simulink model "EKF_Sim_FAEKF"  (R2018a)
settings: Solver=ode4  StartTime=time_start  StopTime=time_end  FixedStep=time_step  MaxStep=0.1  RelTol=1e-6  AbsTol=1e-6
values from neighbouring files (symbols this model uses):
  FUZZY_props =     [FAEKF_FuzzyProps.mat]    (also in FFNAV_FAEKF_RunSim.m = FFNAV_FAEKF_FuzzyInitialize(MSFplot_flag))
  GPS_r_STD = 10*GPS_r_STD    [FFNAV_FAEKF_RunSim.m]
  GPS_v_STD = 10*GPS_v_STD    [FFNAV_FAEKF_RunSim.m]
  N_window = 30    [FFNAV_FAEKF_RunSim.m]
  Q0 = 10*Q0    [FFNAV_FAEKF_RunSim.m]
  Q_adapt = Q0    [FFNAV_FAEKF_FuzzyAdapt.m]    (also in FFNAV_FAEKF_RunSim.m = 0)
  R0 = R0    [FFNAV_FAEKF_RunSim.m]
  R_adapt = R0*beta^(-2*(k))    [FFNAV_FAEKF_FuzzyAdapt.m]    (also in FFNAV_FAEKF_RunSim.m = 0)
  time_step = 1    [FFNAV_FAEKF_RunSim.m]
undefined symbols (not defined in the file or in its folder): COE_chaser, COE_target, Constants, mu, n, PropOptions_chaser, PropOptions_target, theta0_target
libraries: dspindex x9, dspstat3 x7, dspmtrx3 x1
(part 1 of 2)
settings Model: Creator=corytfraser  LastModifiedBy=Cory
settings SolverCC: AutoScaleAbsTol=off
settings DataIOCC: LimitDataPoints=on  SaveFormat=Array  SignalLoggingSaveFormat=ModelDataLogs
settings OptimizationCC: BlockReduction=off  BooleanDataType=off  ExpressionDepthLimit=2147483647  LifeSpan=inf
settings DebuggingCC: SaveWithParameterizedLinksMsg=none  UnderspecifiedInitializationDetection=Classic  MergeDetectMultiDrivingBlocksExec=none  MultiTaskDSMMsg=warning  MultiTaskCondExecSysMsg=none  FcnCallInpInsideContextMsg=warning  AllowSymbolicDim=off  StateNameClashWarn=warning  SFUnexpectedBacktrackingDiag=warning  SFNoUnconditionalDefaultTransitionDiag=warning  SFExecutionAtInitializationDiag=none
settings HardwareCC: ProdBitPerPointer=32  ProdBitPerSizeT=32  ProdBitPerPtrDiffT=32  ProdLargestAtomicFloat=None  ProdIntDivRoundTo=Undefined  ProdEndianess=Unspecified  ProdWordSize=32  ProdHWDeviceType=32-bit Generic  TargetUnknown=on
settings ModelReferenceCC: PropagateSignalLabelsOutOfModel=off
settings CodeAppCC: StateflowObjectComments=on
settings GRTTargetCC: TargetLangStandard=C89/C90 (ANSI)  GeneratePreprocessorConditionals=Disable all
settings ConfigComp: CovMetricSettings=dw  CovHtmlReporting=on  CovSaveCumulativeToWorkspaceVar=on  CovSaveSingleToWorkspaceVar=on  CovExternalEMLEnable=off  CovSFcnEnable=off

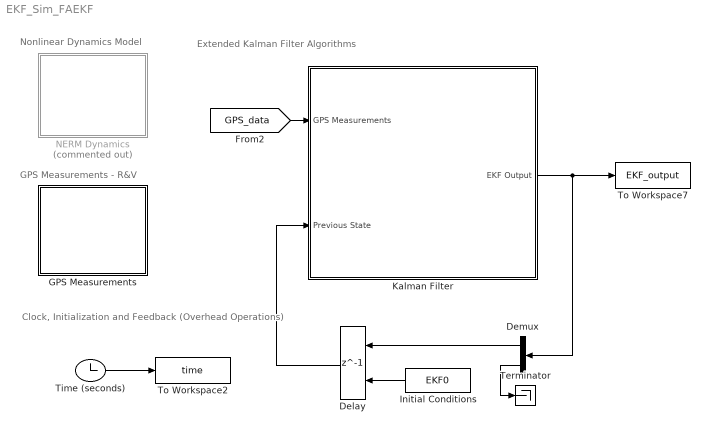
== system EKF_Sim_FAEKF ==
  note: Clock, Initialization and Feedback
      |         (Overhead Operations)
  note: Extended Kalman Filter
      |          Algorithms
  note: GPS Measurements - R&V
  note: Nonlinear Dynamics Model
  Delay : Delay  DelayLength=1  InitialConditionSource=Input port  InitialCondition=0  SampleTime=time_step
      settings: InputPortMap=u0,p4
  Demux : Demux  Outputs=[117 -1]
  "GPS Measurements " : Subsystem
      mask Display: image('C:\Users\Cory\OneDrive\FFNAV Project\MATLAB Code\NERM EKF Simulation\Masks\GPS Image.jpg');
  Initial Conditions : FromWorkspace  VariableName=EKF0  SampleTime=time_step
  Kalman Filter : Subsystem  Variant=on
  NERM Dynamics : Subsystem  Commented=on
      mask Display: image('C:\Users\Cory\OneDrive\FFNAV Project\MATLAB Code\NERM EKF Simulation\Masks\Proba-3.jpg');
  Terminator : Terminator
  Time (seconds) : Clock
      settings: Decimation=1000
  To Workspace2 : ToWorkspace  VariableName=time  SampleTime=-1
  To Workspace7 : ToWorkspace  VariableName=EKF_output  SampleTime=-1
  wires:
  Time (seconds)/1 -> To Workspace2/1
  Kalman Filter/1(EKF Output) -> Demux/1, To Workspace7/1
  Initial Conditions/1 -> Delay/2
  Delay/1 -> Kalman Filter/2(Previous State)
  [GPS_data] -> Kalman Filter/1(GPS Measurements)
  Demux/2 -> Terminator/1
  Demux/1 -> Delay/1

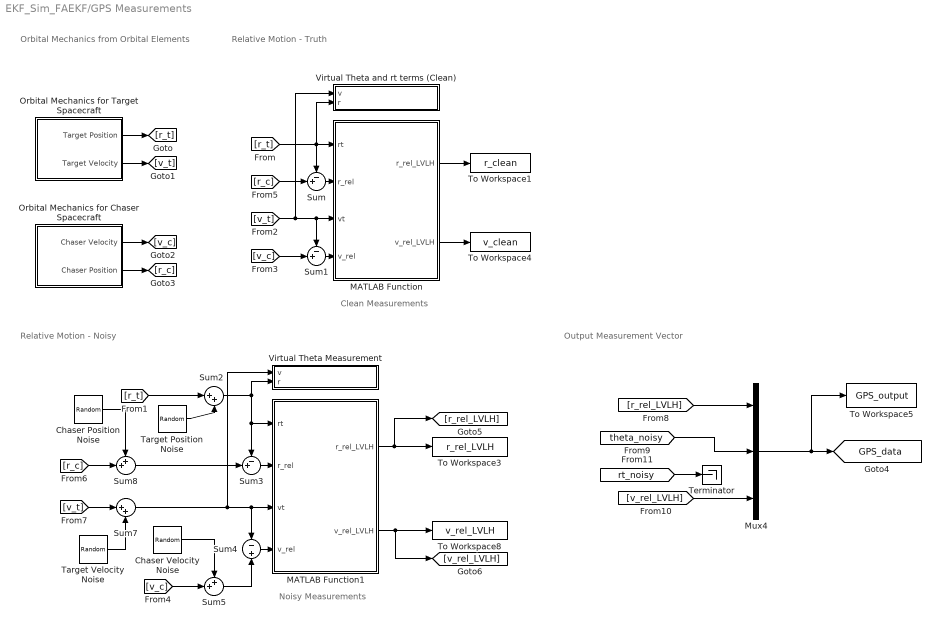
== system EKF_Sim_FAEKF/GPS Measurements  ==
  note: Output Measurement Vector
  note: Relative Motion - Noisy
  note: Relative Motion - Truth
  note: Orbital Mechanics
      | from Orbital Elements
  note: Noisy Measurements
  note: Clean Measurements
  Chaser Position Noise : RandomNumber  Variance=GPS_r_STD^2  Seed=1222  SampleTime=time_step
  Chaser Velocity Noise : RandomNumber  Variance=GPS_v_STD^2  Seed=99999999  SampleTime=time_step
  MATLAB Function : MATLAB Function  TreatAsAtomicUnit=on
  MATLAB Function1 : MATLAB Function  TreatAsAtomicUnit=on
  Mux4 : Mux  Inputs=3
  Orbital Mechanics for Target Spacecraft : Subsystem
  Orbital Mechanics for Chaser Spacecraft : Subsystem
  Sum : Sum  Inputs=-+|
  Sum1 : Sum  Inputs=-+|
  Sum2 : Sum  Inputs=|++
  Sum3 : Sum  Inputs=-+|
  Sum4 : Sum  Inputs=-|+
  Sum5 : Sum  Inputs=++|
  Sum7 : Sum  Inputs=|++
  Sum8 : Sum  Inputs=++|
  Target Position Noise : RandomNumber  Variance=GPS_r_STD^2  Seed=999  SampleTime=time_step
  Target Velocity Noise : RandomNumber  Variance=GPS_v_STD^2  Seed=2000  SampleTime=time_step
  Terminator : Terminator
  To Workspace1 : ToWorkspace  VariableName=r_clean  SampleTime=-1
  To Workspace3 : ToWorkspace  VariableName=r_rel_LVLH  SampleTime=-1
  To Workspace4 : ToWorkspace  VariableName=v_clean  SampleTime=-1
  To Workspace5 : ToWorkspace  VariableName=GPS_output  SampleTime=-1
  To Workspace8 : ToWorkspace  VariableName=v_rel_LVLH  SampleTime=-1
  Virtual Theta Measurement : Subsystem
  Virtual Theta and rt terms (Clean) : Subsystem
  tag scope: GPS_data=global
  wires:
  Orbital Mechanics for Target Spacecraft/1(Target Position) -> [r_t]
  Sum/1 -> MATLAB Function/2(r_rel)
  Sum1/1 -> MATLAB Function/4(v_rel)
  MATLAB Function/2(v_rel_LVLH) -> To Workspace4/1
  MATLAB Function/1(r_rel_LVLH) -> To Workspace1/1
  Mux4/1 -> To Workspace5/1, [GPS_data]
  MATLAB Function1/2(v_rel_LVLH) -> [v_rel_LVLH], To Workspace8/1
  MATLAB Function1/1(r_rel_LVLH) -> [r_rel_LVLH], To Workspace3/1
  Sum7/1 -> Virtual Theta Measurement/1(v), MATLAB Function1/3(vt), Sum4/1
  Sum3/1 -> MATLAB Function1/2(r_rel)
  Sum4/1 -> MATLAB Function1/4(v_rel)
  Sum5/1 -> Sum4/2
  Sum8/1 -> Sum3/2
  [r_t] -> Virtual Theta and rt terms (Clean)/2(r), Sum/1, MATLAB Function/1(rt)
  [v_t] -> Sum1/1, MATLAB Function/3(vt), Virtual Theta and rt terms (Clean)/1(v)
  [v_c] -> Sum1/2
  Orbital Mechanics for Chaser Spacecraft/1(Chaser Velocity) -> [v_c]
  [r_c] -> Sum/2
  Orbital Mechanics for Chaser Spacecraft/2(Chaser Position) -> [r_c]
  Orbital Mechanics for Target Spacecraft/2(Target Velocity) -> [v_t]
  [r_t] -> Sum2/1
  [r_c] -> Sum8/2
  [v_t] -> Sum7/1
  [v_c] -> Sum5/2
  Sum2/1 -> MATLAB Function1/1(rt), Sum3/1, Virtual Theta Measurement/2(r)
  Chaser Position Noise/1 -> Sum8/1
  Target Position Noise/1 -> Sum2/2
  Target Velocity Noise/1 -> Sum7/2
  Chaser Velocity Noise/1 -> Sum5/1
  [r_rel_LVLH] -> Mux4/1
  [v_rel_LVLH] -> Mux4/3
  [theta_noisy] -> Mux4/2
  [rt_noisy] -> Terminator/1

== system EKF_Sim_FAEKF/Kalman Filter ==
  GPS Measurements : Inport
  Previous State : Inport  Port=2
  EKF : Subsystem  VariantControl=EKF_flag == 0
  FAEKF : Subsystem  VariantControl=EKF_flag == 2
  MLE-EKF : Subsystem  VariantControl=EKF_flag == 1
  EKF Output : Outport

== system EKF_Sim_FAEKF/NERM Dynamics ==
  Demux : Demux  Outputs=[10 -1]
  Demux1 : Demux  Outputs=10
  Initial Conditions : FromWorkspace  VariableName=EKF0  SampleTime=time_step
  Mux : Mux  Inputs=10
  NERM Propagation : Subsystem
  Terminator1 : Terminator
  To Workspace6 : ToWorkspace  VariableName=NERM_output  SampleTime=-1
  wires:
  Demux1/9 -> NERM Propagation/9(theta_dot0)
  Demux1/6 -> NERM Propagation/6(x_dot0_chaser)
  Demux1/4 -> NERM Propagation/4(theta0_target)
  Demux1/3 -> NERM Propagation/3(z0_chaser)
  Initial Conditions/1 -> Demux/1
  Demux1/7 -> NERM Propagation/7(y_dot0_chaser)
  Demux1/2 -> NERM Propagation/2(y0_chaser)
  Demux1/1 -> NERM Propagation/1(x0_chaser)
  NERM Propagation/1(x) -> Mux/1
  NERM Propagation/2(y) -> Mux/2
  NERM Propagation/3(z) -> Mux/3
  Demux/1 -> Demux1/1  "Initial  State Vector"
  NERM Propagation/7(y_dot) -> Mux/7
  NERM Propagation/4(theta_target) -> Mux/4
  NERM Propagation/9(theta_dot_target) -> Mux/9
  NERM Propagation/10(rt_dot) -> Mux/10
  NERM Propagation/6(x_dot) -> Mux/6
  NERM Propagation/8(z_dot) -> Mux/8
  NERM Propagation/5(rt) -> Mux/5
  Demux1/8 -> NERM Propagation/8(z_dot0_chaser)
  Mux/1 -> To Workspace6/1
  Demux/2 -> Terminator1/1
  Demux1/5 -> NERM Propagation/5(rt0)
  Demux1/10 -> NERM Propagation/10(rt_dot0)

== system EKF_Sim_FAEKF/GPS Measurements /Orbital Mechanics for Target Spacecraft ==
  Integrator : Integrator  InitialConditionSource=external
  Integrator1 : Integrator  InitialConditionSource=external
  MATLAB Function1 : MATLAB Function  TreatAsAtomicUnit=on
  Target Orbital Mechanics : MATLAB Function  TreatAsAtomicUnit=on
  To Workspace1 : ToWorkspace  VariableName=r_target_ECI  SampleTime=-1
  To Workspace2 : ToWorkspace  VariableName=v_target_ECI  SampleTime=-1
  Target Position : Outport
  Target Velocity : Outport  Port=2
  wires:
  Integrator/1 -> MATLAB Function1/2(V_Sat), To Workspace2/1, Target Velocity/1, Integrator1/1  "r_dot"
  MATLAB Function1/1(r_ddot) -> Integrator/1  "r_ddot"
  Integrator1/1 -> MATLAB Function1/1(R_Sat), To Workspace1/1, Target Position/1  "r"
  Target Orbital Mechanics/2(r_ECI) -> Integrator1/2
  Target Orbital Mechanics/1(v_ECI) -> Integrator/2  "V0"

== system EKF_Sim_FAEKF/GPS Measurements /Orbital Mechanics for Chaser Spacecraft ==
  Integrator : Integrator  InitialConditionSource=external
  Integrator1 : Integrator  InitialConditionSource=external
  MATLAB Function1 : MATLAB Function  TreatAsAtomicUnit=on
  Orbital Mechanics : MATLAB Function  TreatAsAtomicUnit=on
  To Workspace1 : ToWorkspace  VariableName=r_chaser_ECI  SampleTime=-1
  To Workspace2 : ToWorkspace  VariableName=v_chaser_ECI  SampleTime=-1
  Chaser Velocity : Outport
  Chaser Position : Outport  Port=2
  wires:
  Integrator/1 -> MATLAB Function1/2(V_Sat), To Workspace2/1, Chaser Velocity/1, Integrator1/1  "r_dot"
  MATLAB Function1/1(r_ddot) -> Integrator/1  "r_ddot"
  Integrator1/1 -> To Workspace1/1, MATLAB Function1/1(R_Sat), Chaser Position/1  "r"
  Orbital Mechanics/2(r_ECI) -> Integrator1/2
  Orbital Mechanics/1(v_ECI) -> Integrator/2  "V0"

== system EKF_Sim_FAEKF/GPS Measurements /Virtual Theta Measurement ==
  v : Inport
  r : Inport  Port=2
  Integrator2 : Integrator  InitialCondition=theta0_target
  MATLAB Function2 : MATLAB Function  TreatAsAtomicUnit=on
  To Workspace5 : ToWorkspace  VariableName=theta_target  SampleTime=-1
  tag scope: rt_noisy=global, theta_noisy=global
  wires:
  r/1 -> MATLAB Function2/1(r)
  Integrator2/1 -> [theta_noisy], To Workspace5/1
  MATLAB Function2/1(theta_dot) -> Integrator2/1
  v/1 -> MATLAB Function2/2(v)
  MATLAB Function2/2(rt) -> [rt_noisy]

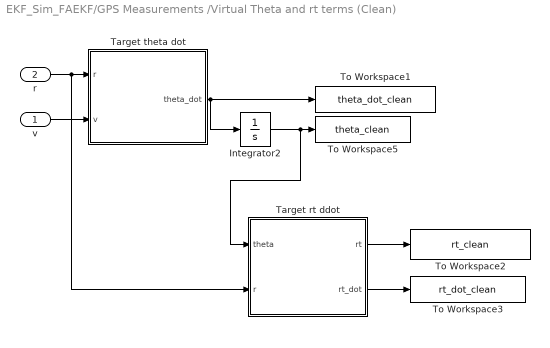
== system EKF_Sim_FAEKF/GPS Measurements /Virtual Theta and rt terms (Clean) ==
  v : Inport
  r : Inport  Port=2
  Integrator2 : Integrator  InitialCondition=theta0_target
  Target rt ddot : MATLAB Function  Tag=hjk  TreatAsAtomicUnit=on
  Target theta dot : MATLAB Function  TreatAsAtomicUnit=on
  To Workspace1 : ToWorkspace  VariableName=theta_dot_clean  SampleTime=-1
  To Workspace2 : ToWorkspace  VariableName=rt_clean  SampleTime=-1
  To Workspace3 : ToWorkspace  VariableName=rt_dot_clean  SampleTime=-1
  To Workspace5 : ToWorkspace  VariableName=theta_clean  SampleTime=-1
  wires:
  r/1 -> Target rt ddot/2(r), Target theta dot/1(r)
  Integrator2/1 -> Target rt ddot/1(theta), To Workspace5/1
  Target theta dot/1(theta_dot) -> Integrator2/1, To Workspace1/1
  v/1 -> Target theta dot/2(v)
  Target rt ddot/1(rt) -> To Workspace2/1
  Target rt ddot/2(rt_dot) -> To Workspace3/1

== system EKF_Sim_FAEKF/Kalman Filter/EKF ==
  Previous State : Inport
  GPS Measurements : Inport  Port=2
  Constant : Constant  Value=Q0
  Constant1 : Constant  Value=R0
  EKF Correction : Subsystem
  EKF Propagation : Subsystem
  To Workspace1 : ToWorkspace  VariableName=R_output  SampleTime=-1
  To Workspace2 : ToWorkspace  VariableName=Q_output  SampleTime=-1
  EKF Output : Outport
  wires:
  Previous State/1 -> EKF Propagation/2(Previous State)
  GPS Measurements/1 -> EKF Correction/3(Sensor Data)
  EKF Propagation/1(Priori state) -> EKF Correction/2(Priori State)
  EKF Correction/1(Posteriori state) -> EKF Output/1
  Constant/1 -> To Workspace2/1, EKF Propagation/1(Q Covariances)
  Constant1/1 -> To Workspace1/1, EKF Correction/1(R Covariances)

== system EKF_Sim_FAEKF/Kalman Filter/FAEKF ==
  note: Extended Kalman Filter
  note: Fuzzy Logic Controller
  Previous State : Inport
  GPS Measurements : Inport  Port=2
  Adaptations : Subsystem
  EKF Correction : Subsystem
  EKF Propagation : Subsystem
  EKF Output : Outport
  wires:
  Previous State/1 -> EKF Propagation/2(Previous State)
  EKF Correction/1(Posteriori state) -> EKF Output/1, Adaptations/1(Previous State)
  Adaptations/1(Adapted Q) -> EKF Propagation/1(Q Covariances)
  Adaptations/2(Adapted R) -> EKF Correction/1(R Covariances)
  EKF Propagation/1(Priori state) -> EKF Correction/2(Priori State)
  GPS Measurements/1 -> EKF Correction/3(Sensor Data)

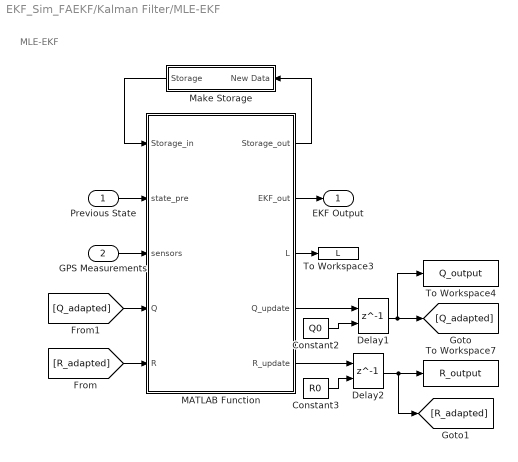
== system EKF_Sim_FAEKF/Kalman Filter/MLE-EKF ==
  note: MLE-EKF
  Previous State : Inport
  GPS Measurements : Inport  Port=2
  Constant2 : Constant  Value=Q0
  Constant3 : Constant  Value=R0
  Delay1 : Delay  DelayLength=1  InitialConditionSource=Input port  InitialCondition=0  SampleTime=time_step
      settings: InputPortMap=u0,p4
  Delay2 : Delay  DelayLength=1  InitialConditionSource=Input port  InitialCondition=0  SampleTime=time_step
      settings: InputPortMap=u0,p4
  MATLAB Function : MATLAB Function  TreatAsAtomicUnit=on
  Make Storage : Subsystem
  To Workspace3 : ToWorkspace  VariableName=L  SampleTime=-1
  To Workspace4 : ToWorkspace  VariableName=Q_output  SampleTime=-1
  To Workspace7 : ToWorkspace  VariableName=R_output  SampleTime=-1
  EKF Output : Outport
  wires:
  MATLAB Function/2(EKF_out) -> EKF Output/1
  MATLAB Function/3(L) -> To Workspace3/1
  MATLAB Function/1(Storage_out) -> Make Storage/1(New Data)
  Make Storage/1(Storage) -> MATLAB Function/1(Storage_in)
  GPS Measurements/1 -> MATLAB Function/3(sensors)
  Previous State/1 -> MATLAB Function/2(state_pre)
  Constant3/1 -> Delay2/2
  Delay2/1 -> To Workspace7/1, [R_adapted]
  MATLAB Function/5(R_update) -> Delay2/1
  [Q_adapted] -> MATLAB Function/4(Q)
  [R_adapted] -> MATLAB Function/5(R)
  Constant2/1 -> Delay1/2
  MATLAB Function/4(Q_update) -> Delay1/1
  Delay1/1 -> To Workspace4/1, [Q_adapted]

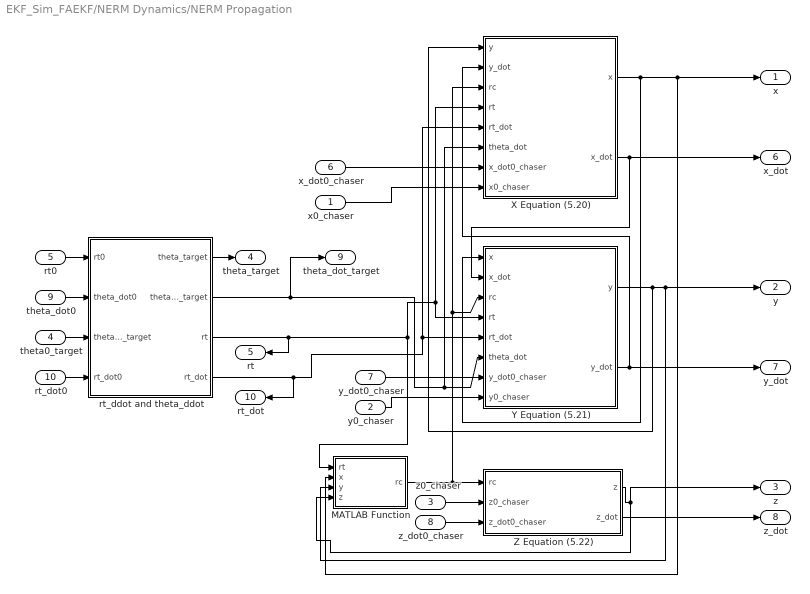
== system EKF_Sim_FAEKF/NERM Dynamics/NERM Propagation ==
  x0_chaser : Inport
  y0_chaser : Inport  Port=2
  z0_chaser : Inport  Port=3
  theta0_target : Inport  Port=4
  rt0 : Inport  Port=5
  x_dot0_chaser : Inport  Port=6
  y_dot0_chaser : Inport  Port=7
  z_dot0_chaser : Inport  Port=8
  theta_dot0 : Inport  Port=9
  rt_dot0 : Inport  Port=10
  MATLAB Function : MATLAB Function  TreatAsAtomicUnit=on
  X Equation (5.20) : Subsystem
  Y Equation (5.21) : Subsystem
  Z Equation (5.22) : Subsystem
  rt_ddot and theta_ddot : Subsystem
  x : Outport
  y : Outport  Port=2
  z : Outport  Port=3
  theta_target : Outport  Port=4
  rt : Outport  Port=5
  x_dot : Outport  Port=6
  y_dot : Outport  Port=7
  z_dot : Outport  Port=8
  theta_dot_target : Outport  Port=9
  rt_dot : Outport  Port=10
  wires:
  MATLAB Function/1(rc) -> X Equation (5.20)/3(rc), Y Equation (5.21)/3(rc), Z Equation (5.22)/1(rc)
  rt_ddot and theta_ddot/4(rt_dot) -> X Equation (5.20)/5(rt_dot), Y Equation (5.21)/5(rt_dot), rt_dot/1
  Y Equation (5.21)/2(y_dot) -> y_dot/1, X Equation (5.20)/2(y_dot)
  X Equation (5.20)/2(x_dot) -> x_dot/1, Y Equation (5.21)/2(x_dot)
  rt_ddot and theta_ddot/2(theta_dot_target) -> theta_dot_target/1, X Equation (5.20)/6(theta_dot), Y Equation (5.21)/6(theta_dot)
  rt_ddot and theta_ddot/3(rt) -> Y Equation (5.21)/4(rt), X Equation (5.20)/4(rt), MATLAB Function/1(rt), rt/1
  X Equation (5.20)/1(x) -> x/1, MATLAB Function/2(x), Y Equation (5.21)/1(x)
  Y Equation (5.21)/1(y) -> y/1, MATLAB Function/3(y), X Equation (5.20)/1(y)
  Z Equation (5.22)/1(z) -> MATLAB Function/4(z), z/1
  rt0/1 -> rt_ddot and theta_ddot/1(rt0)
  theta_dot0/1 -> rt_ddot and theta_ddot/2(theta_dot0)
  y_dot0_chaser/1 -> Y Equation (5.21)/7(y_dot0_chaser)
  y0_chaser/1 -> Y Equation (5.21)/8(y0_chaser)
  x0_chaser/1 -> X Equation (5.20)/8(x0_chaser)
  x_dot0_chaser/1 -> X Equation (5.20)/7(x_dot0_chaser)
  z0_chaser/1 -> Z Equation (5.22)/2(z0_chaser)
  z_dot0_chaser/1 -> Z Equation (5.22)/3(z_dot0_chaser)
  theta0_target/1 -> rt_ddot and theta_ddot/3(theta0_target)
  rt_dot0/1 -> rt_ddot and theta_ddot/4(rt_dot0)
  Z Equation (5.22)/2(z_dot) -> z_dot/1
  rt_ddot and theta_ddot/1(theta_target) -> theta_target/1

== system EKF_Sim_FAEKF/Kalman Filter/EKF/EKF Correction ==
  R Covariances : Inport
  Priori State : Inport  Port=2
  Sensor Data : Inport  Port=3
  MATLAB Function : MATLAB Function  TreatAsAtomicUnit=on
  Posteriori state : Outport
  wires:
  MATLAB Function/1(output) -> Posteriori state/1
  Sensor Data/1 -> MATLAB Function/1(sensors)
  Priori State/1 -> MATLAB Function/2(state_priori)
  R Covariances/1 -> MATLAB Function/3(R)

== system EKF_Sim_FAEKF/Kalman Filter/EKF/EKF Propagation ==
  Q Covariances : Inport
  Previous State : Inport  Port=2
  MATLAB Function : MATLAB Function  TreatAsAtomicUnit=on
  Priori state : Outport
  wires:
  MATLAB Function/1(output) -> Priori state/1
  Previous State/1 -> MATLAB Function/1(state_pre)
  Q Covariances/1 -> MATLAB Function/2(Q)

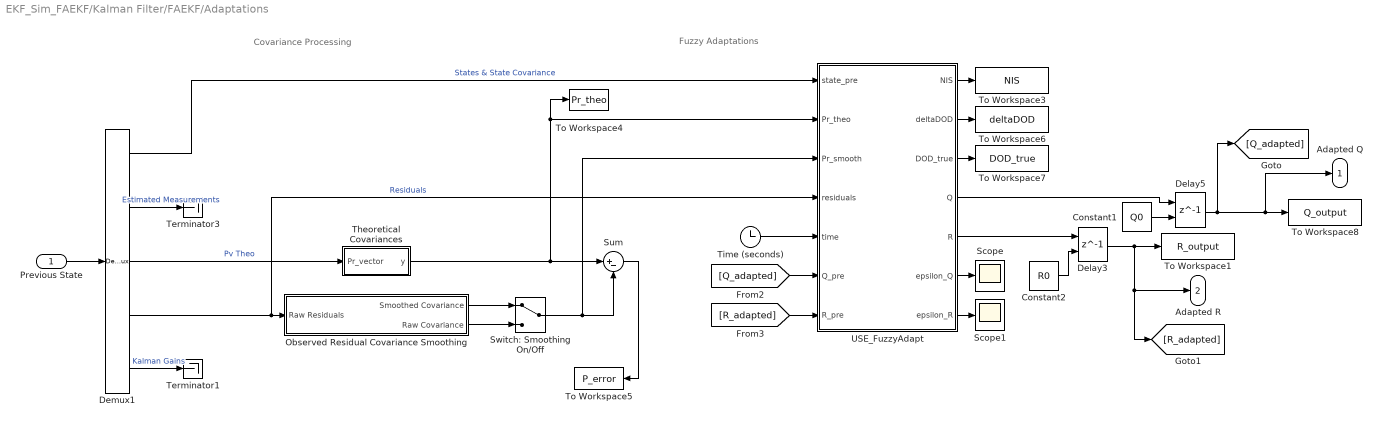
== system EKF_Sim_FAEKF/Kalman Filter/FAEKF/Adaptations ==
  note: Fuzzy Adaptations
  note: Covariance Processing
  Previous State : Inport
  Constant1 : Constant  Value=Q0
  Constant2 : Constant  Value=R0
  Delay3 : Delay  DelayLength=1  InitialConditionSource=Input port  InitialCondition=0  SampleTime=time_step
      settings: InputPortMap=u0,p4
  Delay5 : Delay  DelayLength=1  InitialConditionSource=Input port  InitialCondition=0  SampleTime=time_step
      settings: InputPortMap=u0,p4
  Demux1 : Demux  Outputs="[110 7  49 7 70 ]"
  Observed Residual Covariance Smoothing : Subsystem
  Scope : Scope
  Scope1 : Scope
  Sum : Sum  Inputs=|+-
  Switch: Smoothing On/Off : ManualSwitch
  Terminator1 : Terminator
  Terminator3 : Terminator
  Theoretical Covariances : MATLAB Function  TreatAsAtomicUnit=on
  Time (seconds) : Clock
  To Workspace1 : ToWorkspace  VariableName=R_output  SampleTime=-1
  To Workspace3 : ToWorkspace  VariableName=NIS  SampleTime=-1
  To Workspace4 : ToWorkspace  VariableName=Pr_theo  SampleTime=-1
  To Workspace5 : ToWorkspace  VariableName=P_error  SampleTime=-1
  To Workspace6 : ToWorkspace  VariableName=deltaDOD  SampleTime=-1
  To Workspace7 : ToWorkspace  VariableName=DOD_true  SampleTime=-1
  To Workspace8 : ToWorkspace  VariableName=Q_output  SampleTime=-1
  USE_FuzzyAdapt : MATLAB Function  TreatAsAtomicUnit=on
  Adapted Q : Outport
  Adapted R : Outport  Port=2
  wires:
  Previous State/1 -> Demux1/1
  Theoretical Covariances/1(y) -> USE_FuzzyAdapt/2(Pr_theo), To Workspace4/1, Sum/1
  Demux1/1 -> USE_FuzzyAdapt/1(state_pre)  "States & State Covariance"
  Demux1/2 -> Terminator3/1  "Estimated Measurements"
  Switch: Smoothing On/Off/1 -> Sum/2, USE_FuzzyAdapt/3(Pr_smooth)
  Observed Residual Covariance Smoothing/2(Raw Covariance) -> Switch: Smoothing On/Off/2
  Demux1/3 -> Theoretical Covariances/1(Pr_vector)  "Pv Theo"
  Demux1/4 -> USE_FuzzyAdapt/4(residuals), Observed Residual Covariance Smoothing/1(Raw Residuals)  "Residuals"
  Observed Residual Covariance Smoothing/1(Smoothed Covariance) -> Switch: Smoothing On/Off/1
  Demux1/5 -> Terminator1/1  "Kalman Gains"
  Time (seconds)/1 -> USE_FuzzyAdapt/5(time)
  Sum/1 -> To Workspace5/1
  USE_FuzzyAdapt/1(NIS) -> To Workspace3/1
  USE_FuzzyAdapt/2(deltaDOD) -> To Workspace6/1
  USE_FuzzyAdapt/3(DOD_true) -> To Workspace7/1
  USE_FuzzyAdapt/6(epsilon_Q) -> Scope/1
  USE_FuzzyAdapt/7(epsilon_R) -> Scope1/1
  Constant1/1 -> Delay5/2
  Constant2/1 -> Delay3/2
  [Q_adapted] -> USE_FuzzyAdapt/6(Q_pre)
  [R_adapted] -> USE_FuzzyAdapt/7(R_pre)
  USE_FuzzyAdapt/4(Q) -> Delay5/1
  Delay5/1 -> To Workspace8/1, Adapted Q/1, [Q_adapted]
  USE_FuzzyAdapt/5(R) -> Delay3/1
  Delay3/1 -> [R_adapted], Adapted R/1, To Workspace1/1

== system EKF_Sim_FAEKF/Kalman Filter/FAEKF/EKF Correction ==
  R Covariances : Inport
  Priori State : Inport  Port=2
  Sensor Data : Inport  Port=3
  MATLAB Function : MATLAB Function  TreatAsAtomicUnit=on
  Posteriori state : Outport
  wires:
  MATLAB Function/1(output) -> Posteriori state/1
  Sensor Data/1 -> MATLAB Function/1(sensors)
  Priori State/1 -> MATLAB Function/2(input_priori)
  R Covariances/1 -> MATLAB Function/3(R)

== system EKF_Sim_FAEKF/Kalman Filter/FAEKF/EKF Propagation ==
  Q Covariances : Inport
  Previous State : Inport  Port=2
  MATLAB Function : MATLAB Function  TreatAsAtomicUnit=on
  Priori state : Outport
  wires:
  MATLAB Function/1(output) -> Priori state/1
  Previous State/1 -> MATLAB Function/1(state_pre)
  Q Covariances/1 -> MATLAB Function/2(Q)

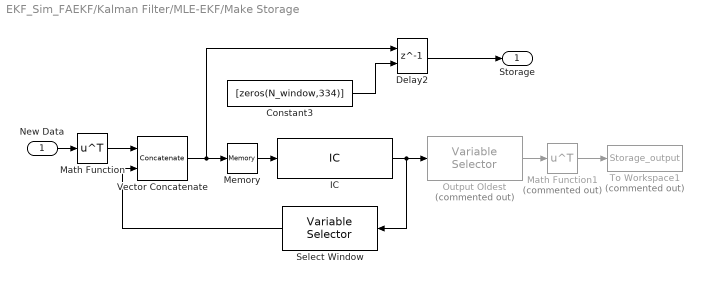
== system EKF_Sim_FAEKF/Kalman Filter/MLE-EKF/Make Storage ==
  New Data : Inport
  Constant3 : Constant  Value=[zeros(N_window,334)]
  Delay2 : Delay  DelayLength=1  InitialConditionSource=Input port  InitialCondition=0  SampleTime=time_step
      settings: InputPortMap=u0,p4
  IC : InitialCondition  Value=[zeros(N_window,334)]
  Math Function : Math  Operator=transpose  SaturateOnIntegerOverflow=on
  Math Function1 : Math  Commented=on  Operator=transpose  SaturateOnIntegerOverflow=on
  Memory : Memory
  Output Oldest : dspindex/Variable Selector  Commented=on  NumInputs=1  rowsOrCols=Rows  IdxMode=Fixed  Elements=N_window  ZerOneIdxMode=One-based  errmode=Clip Index  FillMode=on  FillValues=0
  Select Window : dspindex/Variable Selector  NumInputs=1  rowsOrCols=Rows  IdxMode=Fixed  Elements=1:N_window-1  ZerOneIdxMode=One-based  errmode=Clip Index  FillMode=on  FillValues=0
  To Workspace1 : ToWorkspace  Commented=on  VariableName=Storage_output  SampleTime=-1
  Vector Concatenate : Concatenate  Mode=Multidimensional array
  Storage : Outport
  wires:
  IC/1 -> Output Oldest/1, Select Window/1
  Memory/1 -> IC/1
  Select Window/1 -> Vector Concatenate/2
  New Data/1 -> Math Function/1
  Vector Concatenate/1 -> Delay2/1, Memory/1
  Math Function/1 -> Vector Concatenate/1
  Delay2/1 -> Storage/1
  Constant3/1 -> Delay2/2
  Math Function1/1 -> To Workspace1/1
  Output Oldest/1 -> Math Function1/1

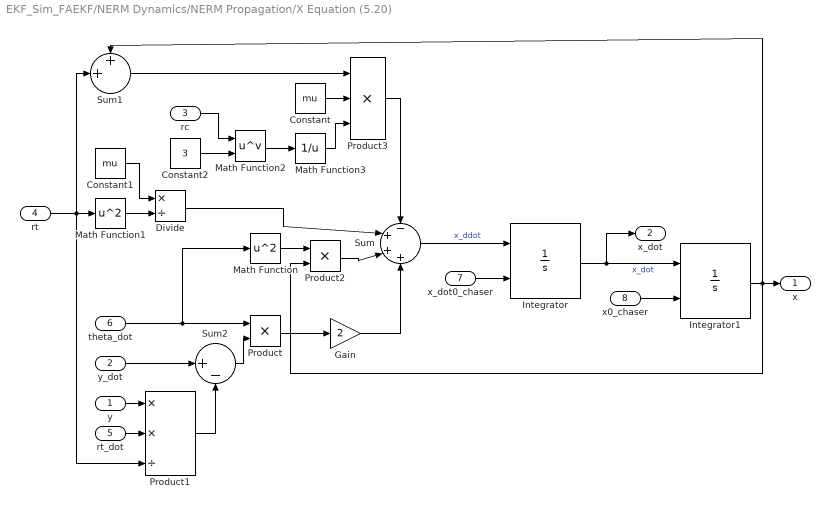
== system EKF_Sim_FAEKF/NERM Dynamics/NERM Propagation/X Equation (5.20) ==
  y : Inport
  y_dot : Inport  Port=2
  rc : Inport  Port=3
  rt : Inport  Port=4
  rt_dot : Inport  Port=5
  theta_dot : Inport  Port=6
  x_dot0_chaser : Inport  Port=7
  x0_chaser : Inport  Port=8
  Constant : Constant  Value=mu
  Constant1 : Constant  Value=mu
  Constant2 : Constant  Value=3
  Divide : Product  Inputs=*/
  Gain : Gain  Gain=2
  Integrator : Integrator  InitialConditionSource=external
  Integrator1 : Integrator  InitialConditionSource=external
  Math Function : Math  Operator=square  SaturateOnIntegerOverflow=on
  Math Function1 : Math  Operator=square  SaturateOnIntegerOverflow=on
  Math Function2 : Math  Operator=pow  SaturateOnIntegerOverflow=on
  Math Function3 : Math  Operator=reciprocal  SaturateOnIntegerOverflow=on
  Product : Product
  Product1 : Product  Inputs=**/
  Product2 : Product
  Product3 : Product  Inputs=3
  Sum : Sum  Inputs=-+++
  Sum1 : Sum  Inputs=++|
  Sum2 : Sum  Inputs=|+-
  x : Outport
  x_dot : Outport  Port=2
  wires:
  Sum/1 -> Integrator/1  "x_ddot"
  Integrator/1 -> Integrator1/1, x_dot/1  "x_dot"
  x_dot0_chaser/1 -> Integrator/2
  Constant/1 -> Product3/2
  Integrator1/1 -> Product2/2, Sum1/1, x/1
  rc/1 -> Math Function2/1
  x0_chaser/1 -> Integrator1/2
  rt/1 -> Sum1/2, Product1/3, Math Function1/1
  Sum1/1 -> Product3/1
  Constant1/1 -> Divide/1
  Divide/1 -> Sum/2
  Product/1 -> Gain/1
  theta_dot/1 -> Product/1, Math Function/1
  y_dot/1 -> Sum2/1
  y/1 -> Product1/1
  rt_dot/1 -> Product1/2
  Product1/1 -> Sum2/2
  Sum2/1 -> Product/2
  Math Function/1 -> Product2/1
  Product2/1 -> Sum/3
  Gain/1 -> Sum/4
  Math Function1/1 -> Divide/2
  Constant2/1 -> Math Function2/2
  Math Function2/1 -> Math Function3/1
  Math Function3/1 -> Product3/3
  Product3/1 -> Sum/1

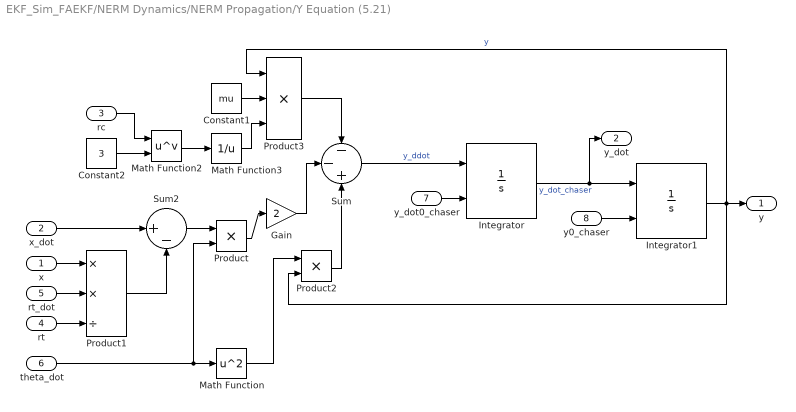
== system EKF_Sim_FAEKF/NERM Dynamics/NERM Propagation/Y Equation (5.21) ==
  x : Inport
  x_dot : Inport  Port=2
  rc : Inport  Port=3
  rt : Inport  Port=4
  rt_dot : Inport  Port=5
  theta_dot : Inport  Port=6
  y_dot0_chaser : Inport  Port=7
  y0_chaser : Inport  Port=8
  Constant1 : Constant  Value=mu
  Constant2 : Constant  Value=3
  Gain : Gain  Gain=2
  Integrator : Integrator  InitialConditionSource=external
  Integrator1 : Integrator  InitialConditionSource=external
  Math Function : Math  Operator=square  SaturateOnIntegerOverflow=on
  Math Function2 : Math  Operator=pow  SaturateOnIntegerOverflow=on
  Math Function3 : Math  Operator=reciprocal  SaturateOnIntegerOverflow=on
  Product : Product
  Product1 : Product  Inputs=**/
  Product2 : Product
  Product3 : Product  Inputs=3
  Sum : Sum  Inputs=--+
  Sum2 : Sum  Inputs=|+-
  y : Outport
  y_dot : Outport  Port=2
  wires:
  y_dot0_chaser/1 -> Integrator/2
  y0_chaser/1 -> Integrator1/2
  Integrator/1 -> y_dot/1, Integrator1/1  "y_dot_chaser"
  Sum/1 -> Integrator/1  "y_ddot"
  Integrator1/1 -> Product2/2, Product3/1, y/1  "y"
  Product/1 -> Gain/1
  theta_dot/1 -> Product/2, Math Function/1
  Product1/1 -> Sum2/2
  Math Function/1 -> Product2/1
  Gain/1 -> Sum/2
  Product2/1 -> Sum/3
  x_dot/1 -> Sum2/1
  x/1 -> Product1/1
  rt_dot/1 -> Product1/2
  rt/1 -> Product1/3
  Sum2/1 -> Product/1
  Constant1/1 -> Product3/2
  rc/1 -> Math Function2/1
  Constant2/1 -> Math Function2/2
  Math Function2/1 -> Math Function3/1
  Math Function3/1 -> Product3/3
  Product3/1 -> Sum/1

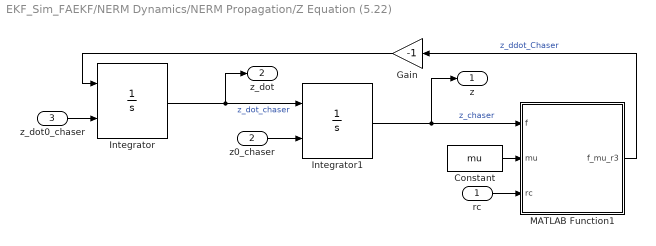
== system EKF_Sim_FAEKF/NERM Dynamics/NERM Propagation/Z Equation (5.22) ==
  rc : Inport
  z0_chaser : Inport  Port=2
  z_dot0_chaser : Inport  Port=3
  Constant : Constant  Value=mu
  Gain : Gain  Gain=-1
  Integrator : Integrator  InitialConditionSource=external
  Integrator1 : Integrator  InitialConditionSource=external
  MATLAB Function1 : MATLAB Function  TreatAsAtomicUnit=on
  z : Outport
  z_dot : Outport  Port=2
  wires:
  Constant/1 -> MATLAB Function1/2(mu)
  Integrator/1 -> z_dot/1, Integrator1/1  "z_dot_chaser"
  Integrator1/1 -> z/1, MATLAB Function1/1(f)  "z_chaser"
  Gain/1 -> Integrator/1
  MATLAB Function1/1(f_mu_r3) -> Gain/1  "z_ddot_Chaser"
  z_dot0_chaser/1 -> Integrator/2
  z0_chaser/1 -> Integrator1/2
  rc/1 -> MATLAB Function1/3(rc)

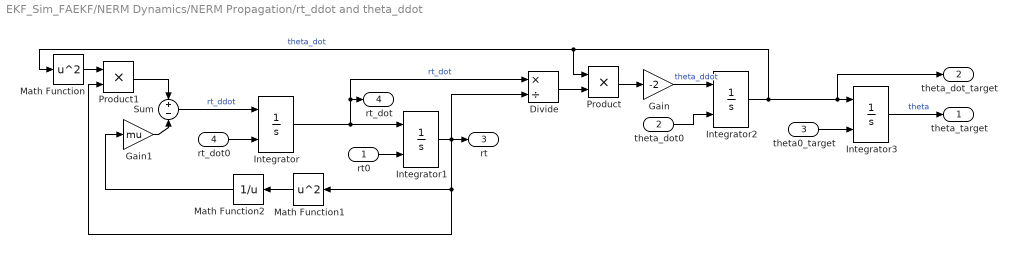
== system EKF_Sim_FAEKF/NERM Dynamics/NERM Propagation/rt_ddot and theta_ddot ==
  rt0 : Inport
  theta_dot0 : Inport  Port=2
  theta0_target : Inport  Port=3
  rt_dot0 : Inport  Port=4
  Divide : Product  Inputs=*/
  Gain : Gain  Gain=-2
  Gain1 : Gain  Gain=mu
  Integrator : Integrator  InitialConditionSource=external
  Integrator1 : Integrator  InitialConditionSource=external
  Integrator2 : Integrator  InitialConditionSource=external  InitialCondition=n
  Integrator3 : Integrator  InitialConditionSource=external
  Math Function : Math  Operator=square  SaturateOnIntegerOverflow=on
  Math Function1 : Math  Operator=square  SaturateOnIntegerOverflow=on
  Math Function2 : Math  Operator=reciprocal  SaturateOnIntegerOverflow=on
  Product : Product
  Product1 : Product
  Sum : Sum  Inputs=+|-
  theta_target : Outport
  theta_dot_target : Outport  Port=2
  rt : Outport  Port=3
  rt_dot : Outport  Port=4
  wires:
  Gain1/1 -> Sum/2
  Math Function2/1 -> Gain1/1
  Math Function1/1 -> Math Function2/1
  Math Function/1 -> Product1/1
  Integrator3/1 -> theta_target/1  "theta"
  Product/1 -> Gain/1
  Sum/1 -> Integrator/1  "rt_ddot"
  Integrator2/1 -> Integrator3/1, theta_dot_target/1, Math Function/1, Product/1  "theta_dot"
  Integrator1/1 -> Product1/2, Math Function1/1, Divide/2, rt/1
  Integrator/1 -> Integrator1/1, Divide/1, rt_dot/1  "rt_dot"
  Divide/1 -> Product/2
  Gain/1 -> Integrator2/1  "theta_ddot"
  theta0_target/1 -> Integrator3/2
  rt_dot0/1 -> Integrator/2
  rt0/1 -> Integrator1/2
  Product1/1 -> Sum/1
  theta_dot0/1 -> Integrator2/2

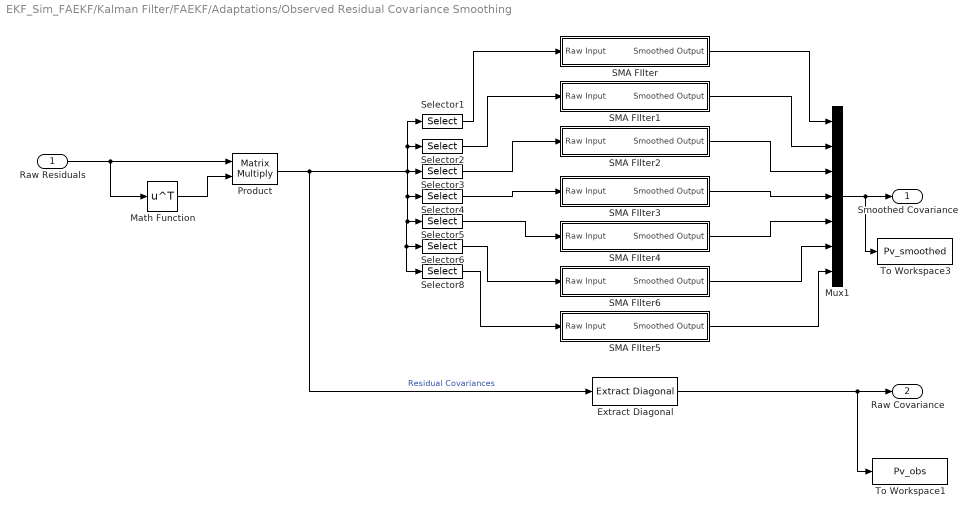
== system EKF_Sim_FAEKF/Kalman Filter/FAEKF/Adaptations/Observed Residual Covariance Smoothing ==
  Raw Residuals : Inport
  Extract Diagonal : dspmtrx3/Extract Diagonal
      settings: SourceProductName=DSP System Toolbox  SourceProductBaseCode=DS
  Math Function : Math  Operator=transpose  SaturateOnIntegerOverflow=on
  Mux1 : Mux  Inputs=7
  Product : Product  Multiplication=Matrix(*)
  SMA FIlter : Subsystem
  SMA FIlter1 : Subsystem
  SMA FIlter2 : Subsystem
  SMA FIlter3 : Subsystem
  SMA FIlter4 : Subsystem
  SMA FIlter5 : Subsystem
  SMA FIlter6 : Subsystem
  Selector1 : Selector  NumberOfDimensions=2  InputPortWidth=3  IndexOptions=Starting index (dialog),Starting index (dialog)  Indices=1,1  OutputSizes=1,1
  Selector2 : Selector  NumberOfDimensions=2  InputPortWidth=3  IndexOptions=Starting index (dialog),Starting index (dialog)  Indices=2,2  OutputSizes=1,1
  Selector3 : Selector  NumberOfDimensions=2  InputPortWidth=3  IndexOptions=Starting index (dialog),Starting index (dialog)  Indices=3,3  OutputSizes=1,1
  Selector4 : Selector  NumberOfDimensions=2  InputPortWidth=3  IndexOptions=Starting index (dialog),Starting index (dialog)  Indices=4,4  OutputSizes=1,1
  Selector5 : Selector  NumberOfDimensions=2  InputPortWidth=3  IndexOptions=Starting index (dialog),Starting index (dialog)  Indices=5,5  OutputSizes=1,1
  Selector6 : Selector  NumberOfDimensions=2  InputPortWidth=3  IndexOptions=Starting index (dialog),Starting index (dialog)  Indices=6,6  OutputSizes=1,1
  Selector8 : Selector  NumberOfDimensions=2  InputPortWidth=3  IndexOptions=Starting index (dialog),Starting index (dialog)  Indices=7,7  OutputSizes=1,1
  To Workspace1 : ToWorkspace  VariableName=Pv_obs  SampleTime=-1
  To Workspace3 : ToWorkspace  VariableName=Pv_smoothed  SampleTime=-1
  Smoothed Covariance : Outport
  Raw Covariance : Outport  Port=2
  wires:
  Selector5/1 -> SMA FIlter4/1(Raw Input)
  SMA FIlter/1(Smoothed Output) -> Mux1/1
  Selector4/1 -> SMA FIlter3/1(Raw Input)
  Selector3/1 -> SMA FIlter2/1(Raw Input)
  Math Function/1 -> Product/2
  SMA FIlter2/1(Smoothed Output) -> Mux1/3
  Product/1 -> Extract Diagonal/1, Selector1/1, Selector2/1, Selector8/1, Selector6/1, Selector5/1, Selector4/1, Selector3/1  "Residual Covariances"
  Raw Residuals/1 -> Math Function/1, Product/1
  SMA FIlter1/1(Smoothed Output) -> Mux1/2
  SMA FIlter3/1(Smoothed Output) -> Mux1/4
  SMA FIlter4/1(Smoothed Output) -> Mux1/5
  SMA FIlter6/1(Smoothed Output) -> Mux1/6
  Selector1/1 -> SMA FIlter/1(Raw Input)
  SMA FIlter5/1(Smoothed Output) -> Mux1/7
  Selector8/1 -> SMA FIlter5/1(Raw Input)
  Selector6/1 -> SMA FIlter6/1(Raw Input)
  Selector2/1 -> SMA FIlter1/1(Raw Input)
  Mux1/1 -> To Workspace3/1, Smoothed Covariance/1
  Extract Diagonal/1 -> To Workspace1/1, Raw Covariance/1

== system EKF_Sim_FAEKF/Kalman Filter/FAEKF/Adaptations/Observed Residual Covariance Smoothing/SMA FIlter ==
  Raw Input : Inport
  IC : InitialCondition  Value=[zeros(N_window,1)]
  Mean : dspstat3/Mean  run=off  InputProcessing=Columns as channels (frame based)  reset_popup=None  directionMode=Each column  dimension=1  roiEnable=off  roiType=Rectangles  roiPortion=Entire ROI  roiOutput=Individual statistics for each ROI  roiFlag=off  roundingMode=Floor  overflowMode=off  outputDataTypeStr=Inherit: Same as accumulator  outputMin=[]  outputMax=[]  outputLastDataTypeStr=Inherit: Same as accumulator
  Memory : Memory
  Mux : Mux  Inputs=2
  Scope : Scope  NumInputPorts=2
  Variable Selector : dspindex/Variable Selector  NumInputs=1  rowsOrCols=Rows  IdxMode=Fixed  Elements=1:N_window-1  ZerOneIdxMode=One-based  errmode=Clip Index  FillMode=on  FillValues=0
  Smoothed Output : Outport
  wires:
  Mux/1 -> Mean/1, Memory/1
  Raw Input/1 -> Scope/1, Mux/1
  Memory/1 -> IC/1
  Variable Selector/1 -> Mux/2
  Mean/1 -> Smoothed Output/1, Scope/2
  IC/1 -> Variable Selector/1

== system EKF_Sim_FAEKF/Kalman Filter/FAEKF/Adaptations/Observed Residual Covariance Smoothing/SMA FIlter1 ==
  Raw Input : Inport
  IC : InitialCondition  Value=[zeros(N_window,1)]
  Mean : dspstat3/Mean  run=off  InputProcessing=Columns as channels (frame based)  reset_popup=None  directionMode=Each column  dimension=1  roiEnable=off  roiType=Rectangles  roiPortion=Entire ROI  roiOutput=Individual statistics for each ROI  roiFlag=off  roundingMode=Floor  overflowMode=off  outputDataTypeStr=Inherit: Same as accumulator  outputMin=[]  outputMax=[]  outputLastDataTypeStr=Inherit: Same as accumulator
  Memory : Memory
  Mux : Mux  Inputs=2
  Scope : Scope  NumInputPorts=2
  Variable Selector : dspindex/Variable Selector  NumInputs=1  rowsOrCols=Rows  IdxMode=Fixed  Elements=1:N_window-1  ZerOneIdxMode=One-based  errmode=Clip Index  FillMode=on  FillValues=0
  Smoothed Output : Outport
  wires:
  Mux/1 -> Mean/1, Memory/1
  Raw Input/1 -> Scope/1, Mux/1
  Memory/1 -> IC/1
  Variable Selector/1 -> Mux/2
  Mean/1 -> Smoothed Output/1, Scope/2
  IC/1 -> Variable Selector/1

== system EKF_Sim_FAEKF/Kalman Filter/FAEKF/Adaptations/Observed Residual Covariance Smoothing/SMA FIlter2 ==
  Raw Input : Inport
  IC : InitialCondition  Value=[zeros(N_window,1)]
  Mean : dspstat3/Mean  run=off  InputProcessing=Columns as channels (frame based)  reset_popup=None  directionMode=Each column  dimension=1  roiEnable=off  roiType=Rectangles  roiPortion=Entire ROI  roiOutput=Individual statistics for each ROI  roiFlag=off  roundingMode=Floor  overflowMode=off  outputDataTypeStr=Inherit: Same as accumulator  outputMin=[]  outputMax=[]  outputLastDataTypeStr=Inherit: Same as accumulator
  Memory : Memory
  Mux : Mux  Inputs=2
  Scope : Scope  NumInputPorts=2
  Variable Selector : dspindex/Variable Selector  NumInputs=1  rowsOrCols=Rows  IdxMode=Fixed  Elements=1:N_window-1  ZerOneIdxMode=One-based  errmode=Clip Index  FillMode=on  FillValues=0
  Smoothed Output : Outport
  wires:
  Mux/1 -> Mean/1, Memory/1
  Raw Input/1 -> Scope/1, Mux/1
  Memory/1 -> IC/1
  Variable Selector/1 -> Mux/2
  Mean/1 -> Smoothed Output/1, Scope/2
  IC/1 -> Variable Selector/1

== system EKF_Sim_FAEKF/Kalman Filter/FAEKF/Adaptations/Observed Residual Covariance Smoothing/SMA FIlter3 ==
  Raw Input : Inport
  IC : InitialCondition  Value=[zeros(N_window,1)]
  Mean : dspstat3/Mean  run=off  InputProcessing=Columns as channels (frame based)  reset_popup=None  directionMode=Each column  dimension=1  roiEnable=off  roiType=Rectangles  roiPortion=Entire ROI  roiOutput=Individual statistics for each ROI  roiFlag=off  roundingMode=Floor  overflowMode=off  outputDataTypeStr=Inherit: Same as accumulator  outputMin=[]  outputMax=[]  outputLastDataTypeStr=Inherit: Same as accumulator
  Memory : Memory
  Mux : Mux  Inputs=2
  Scope : Scope  NumInputPorts=2
  Variable Selector : dspindex/Variable Selector  NumInputs=1  rowsOrCols=Rows  IdxMode=Fixed  Elements=1:N_window-1  ZerOneIdxMode=One-based  errmode=Clip Index  FillMode=on  FillValues=0
  Smoothed Output : Outport
  wires:
  Mux/1 -> Mean/1, Memory/1
  Raw Input/1 -> Scope/1, Mux/1
  Memory/1 -> IC/1
  Variable Selector/1 -> Mux/2
  Mean/1 -> Smoothed Output/1, Scope/2
  IC/1 -> Variable Selector/1

== system EKF_Sim_FAEKF/Kalman Filter/FAEKF/Adaptations/Observed Residual Covariance Smoothing/SMA FIlter4 ==
  Raw Input : Inport
  IC : InitialCondition  Value=[zeros(N_window,1)]
  Mean : dspstat3/Mean  run=off  InputProcessing=Columns as channels (frame based)  reset_popup=None  directionMode=Each column  dimension=1  roiEnable=off  roiType=Rectangles  roiPortion=Entire ROI  roiOutput=Individual statistics for each ROI  roiFlag=off  roundingMode=Floor  overflowMode=off  outputDataTypeStr=Inherit: Same as accumulator  outputMin=[]  outputMax=[]  outputLastDataTypeStr=Inherit: Same as accumulator
  Memory : Memory
  Mux : Mux  Inputs=2
  Scope : Scope  NumInputPorts=2
  Variable Selector : dspindex/Variable Selector  NumInputs=1  rowsOrCols=Rows  IdxMode=Fixed  Elements=1:N_window-1  ZerOneIdxMode=One-based  errmode=Clip Index  FillMode=on  FillValues=0
  Smoothed Output : Outport
  wires:
  Mux/1 -> Mean/1, Memory/1
  Raw Input/1 -> Scope/1, Mux/1
  Memory/1 -> IC/1
  Variable Selector/1 -> Mux/2
  Mean/1 -> Smoothed Output/1, Scope/2
  IC/1 -> Variable Selector/1

== system EKF_Sim_FAEKF/Kalman Filter/FAEKF/Adaptations/Observed Residual Covariance Smoothing/SMA FIlter5 ==
  Raw Input : Inport
  IC : InitialCondition  Value=[zeros(N_window,1)]
  Mean : dspstat3/Mean  run=off  InputProcessing=Columns as channels (frame based)  reset_popup=None  directionMode=Each column  dimension=1  roiEnable=off  roiType=Rectangles  roiPortion=Entire ROI  roiOutput=Individual statistics for each ROI  roiFlag=off  roundingMode=Floor  overflowMode=off  outputDataTypeStr=Inherit: Same as accumulator  outputMin=[]  outputMax=[]  outputLastDataTypeStr=Inherit: Same as accumulator
  Memory : Memory
  Mux : Mux  Inputs=2
  Scope : Scope  NumInputPorts=2
  Variable Selector : dspindex/Variable Selector  NumInputs=1  rowsOrCols=Rows  IdxMode=Fixed  Elements=1:N_window-1  ZerOneIdxMode=One-based  errmode=Clip Index  FillMode=on  FillValues=0
  Smoothed Output : Outport
  wires:
  Mux/1 -> Mean/1, Memory/1
  Raw Input/1 -> Scope/1, Mux/1
  Memory/1 -> IC/1
  Variable Selector/1 -> Mux/2
  Mean/1 -> Smoothed Output/1, Scope/2
  IC/1 -> Variable Selector/1

== system EKF_Sim_FAEKF/Kalman Filter/FAEKF/Adaptations/Observed Residual Covariance Smoothing/SMA FIlter6 ==
  Raw Input : Inport
  IC : InitialCondition  Value=[zeros(N_window,1)]
  Mean : dspstat3/Mean  run=off  InputProcessing=Columns as channels (frame based)  reset_popup=None  directionMode=Each column  dimension=1  roiEnable=off  roiType=Rectangles  roiPortion=Entire ROI  roiOutput=Individual statistics for each ROI  roiFlag=off  roundingMode=Floor  overflowMode=off  outputDataTypeStr=Inherit: Same as accumulator  outputMin=[]  outputMax=[]  outputLastDataTypeStr=Inherit: Same as accumulator
  Memory : Memory
  Mux : Mux  Inputs=2
  Scope : Scope  NumInputPorts=2
  Variable Selector : dspindex/Variable Selector  NumInputs=1  rowsOrCols=Rows  IdxMode=Fixed  Elements=1:N_window-1  ZerOneIdxMode=One-based  errmode=Clip Index  FillMode=on  FillValues=0
  Smoothed Output : Outport
  wires:
  Mux/1 -> Mean/1, Memory/1
  Raw Input/1 -> Scope/1, Mux/1
  Memory/1 -> IC/1
  Variable Selector/1 -> Mux/2
  Mean/1 -> Smoothed Output/1, Scope/2
  IC/1 -> Variable Selector/1

== matlab function EKF_Sim_FAEKF/GPS Measurements /Orbital Mechanics for Target Spacecraft/MATLAB Function1 ==
  data: R_Sat input; V_Sat input; r_ddot output; Constants parameter; PropOptions_target parameter
function r_ddot = r_ddot(R_Sat, V_Sat, Constants, PropOptions_target )
% ========================================================================
% Description: This function calculates -mu/r^3 *r to propagate the radius
% vector of the orbital motion

coder.extrinsic('Accelerations');

r_ddot = zeros(3,1);
r_ddot = Accelerations(R_Sat, V_Sat, Constants, PropOptions_target);

end
% ========================================================================

== matlab function EKF_Sim_FAEKF/GPS Measurements /Orbital Mechanics for Target Spacecraft/Target Orbital Mechanics ==
  data: v_ECI output; r_ECI output; mu parameter; COE_target parameter
 function [v_ECI,r_ECI] = Orb_Mech(mu, COE_target)
% ========================================================================
% Description: This funciton calculates the initial r and v vectors, 
% given the provided classiclal orbital elements defined in the
% initialization of the simulation.

%%========================================================================
%Extract COE values
theta       = COE_target(1);
a           = COE_target(2);
e           = COE_target(3);
i           = COE_target(4);
RAAN        = COE_target(5);
w           = COE_target(6);

%%========================================================================
p   = a*(1-e^2);                                                %Defining the semilatus rectum (Eq. 2.31)
r   = p/(1+e*cos(theta));                               %Defining the radius (Eq. 2.32)

r_P = [r*cos(theta) r*sin(theta) 0]';                           %(r in perifocal frame - Eq. 2.86) 
v_P = [-sqrt(mu/p)*sin(theta) sqrt(mu/p)*(e+cos(theta)) 0]';    %(v in perifocal frame - Eq. 2.87)

%Rotation Matrix from P to ECI Frame
C_IP = [    cos(RAAN)*cos(w)-sin(RAAN)*cos(i)*sin(w) -cos(RAAN)*sin(w)-sin(RAAN)*cos(i)*cos(w) sin(RAAN)*sin(i);
            sin(RAAN)*cos(w)+cos(RAAN)*cos(i)*sin(w) -sin(RAAN)*sin(w)+cos(RAAN)*cos(i)*cos(w) -cos(RAAN)*sin(i);
                        sin(i)*sin(w)                            sin(i)*cos(w)                       cos(i)  ];

%Definition of ECI Frame
x_ECI   = [1 0 0];
y_ECI   = [0 1 0];
z_ECI   = [0 0 1];
F_ECI   = [x_ECI; y_ECI; z_ECI]; %Reference Frame ECI

%r and v vectors in ECI Frame
r_ECI   = F_ECI*C_IP*r_P;
v_ECI   = F_ECI*C_IP*v_P;

%z_vec_ECI  = cross(r_ECI, v_ECI)/norm(cross(r_ECI, v_ECI));    %Check orientation of z vector
%X_ECI      = [r_ECI v_ECI]';                                   %State Vector in ECI components (Eq. 2.82)

r_mag = norm(r_ECI);
r_hat = r_ECI/r_mag;

end
% ========================================================================

== matlab function EKF_Sim_FAEKF/GPS Measurements /Orbital Mechanics for Chaser Spacecraft/MATLAB Function1 ==
  data: R_Sat input; r_ddot output; V_Sat input; Constants parameter; PropOptions_chaser parameter
function r_ddot = r_ddot(R_Sat, V_Sat, Constants, PropOptions_chaser)
% ========================================================================
% Description: This function calculates -mu/r^3 *r to propagate the radius
% vector of the orbital motion

coder.extrinsic('Accelerations');

r_ddot = zeros(3,1);
r_ddot = Accelerations(R_Sat, V_Sat, Constants, PropOptions_chaser);

end
% ========================================================================

== matlab function EKF_Sim_FAEKF/GPS Measurements /Orbital Mechanics for Chaser Spacecraft/Orbital Mechanics ==
  data: v_ECI output; r_ECI output; mu parameter; COE_chaser parameter
function [v_ECI,r_ECI] = Orb_Mech(mu, COE_chaser)
% ========================================================================
% Description: This funciton calculates the initial r and v vectors, 
% given the provided classiclal orbital elements defined in the
% initialization of the simulation.

%%========================================================================
%Extract COE values
theta       = COE_chaser(1);
a           = COE_chaser(2);
e           = COE_chaser(3);
i           = COE_chaser(4);
RAAN        = COE_chaser(5);
w           = COE_chaser(6);

%%========================================================================
p   = a*(1-e^2);                                                %Defining the semilatus rectum (Eq. 31)
r   = p/(1+e*cos(theta));                                       %Defining the radius (Eq. 2.32)
r_P = [r*cos(theta) r*sin(theta) 0]';                           %(r in perifocal frame - Eq. 2.86) 
v_P = [-sqrt(mu/p)*sin(theta) sqrt(mu/p)*(e+cos(theta)) 0]';    %(v in perifocal frame - Eq. 2.87)

%Rotation Matrix from P to ECI Frame
C_IP = [    cos(RAAN)*cos(w)-sin(RAAN)*cos(i)*sin(w) -cos(RAAN)*sin(w)-sin(RAAN)*cos(i)*cos(w) sin(RAAN)*sin(i);
            sin(RAAN)*cos(w)+cos(RAAN)*cos(i)*sin(w) -sin(RAAN)*sin(w)+cos(RAAN)*cos(i)*cos(w) -cos(RAAN)*sin(i);
                        sin(i)*sin(w)                            sin(i)*cos(w)                       cos(i)  ];

%Definition of ECI Frame
x_ECI   = [1 0 0];
y_ECI   = [0 1 0];
z_ECI   = [0 0 1];
F_ECI   = [x_ECI; y_ECI; z_ECI]; %Reference Frame ECI

%r and v vectors in ECI Frame
r_ECI   = F_ECI*C_IP*r_P;
v_ECI   = F_ECI*C_IP*v_P;

%z_vec_ECI  = cross(r_ECI, v_ECI)/norm(cross(r_ECI, v_ECI));    %Check orientation of z vector
%X_ECI      = [r_ECI v_ECI]';                                   %State Vector in ECI components (Eq. 2.82)

r_mag = norm(r_ECI);
r_hat = r_ECI/r_mag;

end
% ========================================================================

== matlab function EKF_Sim_FAEKF/GPS Measurements /MATLAB Function ==
  data: rt input; r_rel input; vt input; r_rel_LVLH output; v_rel input; v_rel_LVLH output
 function [r_rel_LVLH, v_rel_LVLH] = To_LVLH(rt, r_rel, vt, v_rel)
% =========================================================================
% Description: This function converts the relative r and v from ECI Frame
% to LVLH Frame by applying the appropriate rotation matrices.
% =========================================================================
%Determine unit vectors for LVLH Frame
Lx      = rt/norm(rt);
Lz      = cross(rt, vt)/norm(cross(rt, vt));
Ly      = cross(Lz, Lx);

%Align unit vectors into rows
Lx      = Lx';
Ly      = Ly';
Lz      = Lz';

%Arranging vectrix for LVLH Frame
F_LVLH  = [ Lx      
            Ly
            Lz ];

%ECI Frame is defined as such
F_ECI   = [ 1 0 0 
            0 1 0
            0 0 1 ];
     
%Compute roration matrix - ECI to LVLH
C_LI    = F_LVLH*F_ECI';

%Computing relative velocity in LVLH frame, accounting for rotation 
omega =  cross(rt,vt)/norm(rt)^2;
v_rel = v_rel - cross(omega,r_rel);

%Apply rotation to obtain relative LVLH parameters
r_rel_LVLH = C_LI*r_rel; 
v_rel_LVLH = C_LI*v_rel;

end
% =========================================================================

== matlab function EKF_Sim_FAEKF/NERM Dynamics/NERM Propagation/MATLAB Function ==
  data: rt input; x input; y input; z input; rc output
function rc = calc_rc(rt, x, y, z)
% ========================================================================
% Description: This function calculates the radius of the chaser given the
% x, y z and rt components

%Inputs:
%    rt = Target Radius
%    x = Chaser relative x position
%    y = Chaser relative y position
%    z = Chaser relative z position
%Outputs:
%    rc = Chaser Radius

rc = sqrt((rt+x)^2+y^2+z^2);
end
% ========================================================================

== matlab function EKF_Sim_FAEKF/NERM Dynamics/NERM Propagation/Z Equation (5.22)/MATLAB Function1 ==
  data: f input; f_mu_r3 output; mu input; rc input
function f_mu_r3 = mu_rc3(f, mu, rc)
% ========================================================================
% Description: This function calculates mu/rc^3 and multiplies it with the
% incoming signal for the z equation of motion.

f_mu_r3 = (mu/rc^3)*f;
end
% ========================================================================

== matlab function EKF_Sim_FAEKF/GPS Measurements /Virtual Theta Measurement/MATLAB Function2 ==
  data: r input; v input; theta_dot output; rt output
function [theta_dot, rt] = theta_dot(r, v)
% ========================================================================
% Description: This function calculates h/r^2 to propagate the true 
% anomaly of the target spacecraft
rt = norm(r);
h = norm(cross(r,v));
theta_dot = h/rt^2;

end
% ========================================================================

== matlab function EKF_Sim_FAEKF/GPS Measurements /MATLAB Function1 ==
  data: rt input; r_rel input; vt input; r_rel_LVLH output; v_rel input; v_rel_LVLH output
 function [r_rel_LVLH, v_rel_LVLH] = To_LVLH(rt, r_rel, vt, v_rel)
% =========================================================================
% Description: This function converts the relative r and v from ECI Frame
% to LVLH Frame by applying the appropriate rotation matrices.
% =========================================================================
%Determine unit vectors for LVLH Frame
Lx      = rt/norm(rt);
Lz      = cross(rt, vt)/norm(cross(rt, vt));
Ly      = cross(Lz, Lx);

%Align unit vectors into rows
Lx      = Lx';
Ly      = Ly';
Lz      = Lz';

%Arranging vectrix for LVLH Frame
F_LVLH  = [ Lx
            Ly
            Lz ];

%ECI Frame is defined as such
F_ECI   = [ 1 0 0 
            0 1 0
            0 0 1 ];
     
%Compute roration matrix - ECI to LVLH
C_LI    = F_LVLH*F_ECI';

%Computing relative velocity in LVLH frame, accounting for rotation 
omega =  cross(rt,vt)/norm(rt)^2;
v_rel = v_rel - cross(omega,r_rel);

%Apply rotation to obtain relative LVLH parameters
r_rel_LVLH = C_LI*r_rel; 
v_rel_LVLH = C_LI*v_rel;

end
% =========================================================================

== matlab function EKF_Sim_FAEKF/GPS Measurements /Virtual Theta and rt terms (Clean)/Target theta dot ==
  data: r input; v input; theta_dot output
function theta_dot  = theta_dot(r, v)
% ========================================================================
% Description: This function calculates h/r^2 to propagate the true 
% anomaly of the target spacecraft
rt = norm(r);
h = norm(cross(r,v));
theta_dot = h/rt^2;

end
% ========================================================================

== matlab function EKF_Sim_FAEKF/GPS Measurements /Virtual Theta and rt terms (Clean)/Target rt ddot ==
  data: theta input; r input; rt output; rt_dot output; mu parameter; COE_target parameter
function [rt, rt_dot]  = rt_rtdot(theta, r, mu, COE_target)
% ========================================================================
% Description: This function calculates h/r^2 to propagate the true 
% anomaly of the target spacecraft

theta0      = COE_target(1);
SMA         = COE_target(2);
ECC         = COE_target(3);
INC         = COE_target(4);
RAAN        = COE_target(5);
AOP         = COE_target(6);

rt      = norm(r);
p       = SMA*(1-ECC^2);
rt_dot  = sqrt(mu/p)*ECC*sin(theta);

end
% ========================================================================
